simulink model "test_pont_H"  (R2013a)
settings: Solver=ode3  StartTime=0.0  StopTime=1  FixedStep=5e-5  RelTol=1e-3
libraries: powerlib x18, simulink x2, powerlib_meascontrol x2
settings Model: Creator=Daniel  LastModifiedBy=Daniel
settings SolverCC: AlgebraicLoopSolver=LineSearch

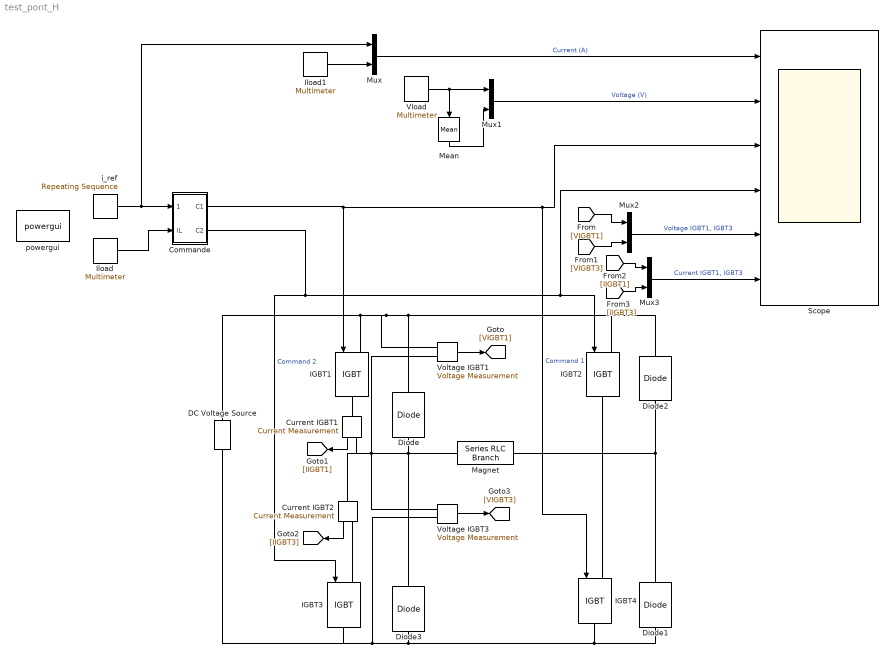
== system test_pont_H ==
  Commande : Subsystem  TreatAsAtomicUnit=on
      settings: MinAlgLoopOccurrences=on
  Current IGBT1 : powerlib/Measurements/Current Measurement  PhasorSimulation=off  OutputType=Complex  PSBequivalent=0
  Current IGBT2 : powerlib/Measurements/Current Measurement  PhasorSimulation=off  OutputType=Complex  PSBequivalent=0
  DC Voltage Source : powerlib/Electrical Sources/DC Voltage Source  Amplitude=5000  Measurements=None
  Diode{,1..3} (4 alike) : powerlib/Power Electronics/Diode  Ron=0.001  Lon=0  Vf=0.8  IC=0  UseSnubber=off  Rs=1  Cs=inf  Measurements=off
  IGBT{1..4} (4 alike) : powerlib/Power Electronics/IGBT  Ron=0.001  Lon=0  Vf=1  Tf=1e-6  Tt=2e-6  IC=0  Rs=0  Cs=0  Measurements=off
  Iload : powerlib/Measurements/Multimeter  PhasorSimulation=off  OutputType=Complex  sel=2  L=2  Gain=1  yselected={'Ib: Magnet '};  PSBOutputType=1  PSBequivalent=0  AxesSetting=[0,0.1,-100,100]  Display=0  SavedBlockNames=-11
  Iload1 : powerlib/Measurements/Multimeter  PhasorSimulation=off  OutputType=Complex  sel=2  L=2  Gain=1  yselected={'Ib: Magnet '};  PSBOutputType=1  PSBequivalent=0  AxesSetting=[0,0.1,-100,100]  Display=0  SavedBlockNames=-11
  "Magnet " : powerlib/Elements/Series RLC Branch  LConnTagsString=__new0  RConnTagsString=__new0  BranchType=RL  Resistance=0.28  Inductance=0.1  SetiL0=off  InitialCurrent=0  Capacitance=1e-6  Setx0=off  InitialVoltage=0  Measurements=Branch voltage and current
  Mean : powerlib_meascontrol/Measurements/Mean  Freq=1e3  Vinit=0  Ts=0
  Mux{,1..3} (4 alike) : Mux  Inputs=2
  Scope : Scope  NumInputPorts=6
      settings: YMin=0~-12500~0~0~-5~-5  YMax=2500~7500~1~1~5~5
  Vload : powerlib/Measurements/Multimeter  PhasorSimulation=off  OutputType=Complex  sel=1  L=2  Gain=1  yselected={'Ub: Magnet '};  PSBOutputType=1  PSBequivalent=0  AxesSetting=[0,0.1,-100,100]  Display=0  SavedBlockNames=-11
  Voltage IGBT1 : powerlib/Measurements/Voltage Measurement  PhasorSimulation=off  OutputType=Complex  PSBequivalent=0
  Voltage IGBT3 : powerlib/Measurements/Voltage Measurement  PhasorSimulation=off  OutputType=Complex  PSBequivalent=0
  "i_ref " : simulink/Sources/Repeating Sequence  rep_seq_t=[0 100e-3 100.1e-3 475e-3 550e-3 708.4e-3 900e-3]  rep_seq_y=[0 0 250 6000 6000 250 250]
  powergui : powerlib/powergui  Priority=1  SimulationMode=Discrete  SolverType=Tustin  SampleTime=50e-6  frequency=60  SPID=off  DisableSnubberDevices=off  DisableRonSwitches=off  DisableVfSwitches=off  SwTol=0  Interpol=off  DisplayEquations=off  frequencyindice=0  Pbase=100e6  ErrMax=1e-4  Iterations=50  UnitsV=kV  UnitsW=MW  FunctionMessages=off  echomessages=off  HookPort=off  EnableUseOfTLC=off  x0status=blocks  RestoreLinks=warning  ResistiveCurrentMeasurement=off  Frange=[0:2:500]  Ylog=off  Xlog=on  ShowGrid=off  save=off  variable=ZData  ZoomFFT=off  StartTime=0.0  cycles=1  DisplayStyle=1  fundamental=60  FreqAxis=off  MaxFrequency=1000  frequencyindicesteady=1  RmsSteady=1  display=off  Ts=0  methode=off
  wires:
  Iload/1 -> Commande/2(IL)
  Commande/1(C1) -> IGBT1/1, IGBT4/1, Scope/3  "Command 1"
  Commande/2(C2) -> IGBT3/1, IGBT2/1, Scope/4  "Command 2"
  Iload1/1 -> Mux/2
  Mux/1 -> Scope/1  "Current (A)"
  Mux1/1 -> Scope/2  "Voltage (V)"
  Vload/1 -> Mean/1, Mux1/1
  Mean/1 -> Mux1/2
  "i_ref "/1 -> Mux/1, Commande/1(Iref)
  Voltage IGBT1/1 -> [VIGBT1]
  Voltage IGBT3/1 -> [VIGBT3]
  [VIGBT1] -> Mux2/1
  [IIGBT1] -> Mux3/1
  [IIGBT3] -> Mux3/2
  Mux2/1 -> Scope/5  "Voltage IGBT1, IGBT3"
  Mux3/1 -> Scope/6  "Current IGBT1, IGBT3"
  Current IGBT1/1 -> [IIGBT1]
  Current IGBT2/1 -> [IIGBT3]
  [VIGBT3] -> Mux2/2
  connections:
  Diode/LConn1 -- Voltage IGBT1/LConn2 -- Current IGBT2/LConn1 -- Current IGBT1/RConn1 -- Voltage IGBT3/LConn1 -- "Magnet "/LConn1 -- Diode3/RConn1
  DC Voltage Source/RConn1 -- IGBT1/LConn1 -- IGBT2/LConn1 -- Diode2/RConn1 -- Diode/RConn1 -- Voltage IGBT1/LConn1
  Diode1/LConn1 -- IGBT4/RConn1 -- Voltage IGBT3/LConn2 -- IGBT3/RConn1 -- DC Voltage Source/LConn1 -- Diode3/LConn1
  Diode1/RConn1 -- Diode2/LConn1 -- IGBT4/LConn1 -- IGBT2/RConn1 -- "Magnet "/RConn1
  IGBT1/RConn1 -- Current IGBT1/LConn1
  IGBT3/LConn1 -- Current IGBT2/RConn1

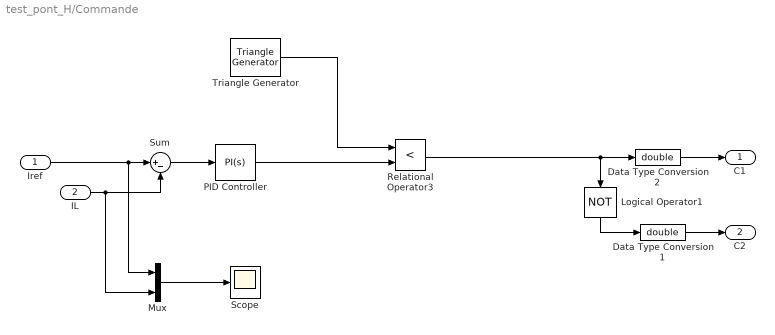
== system test_pont_H/Commande ==
  Iref : Inport
  IL : Inport  Port=2
  Data Type Conversion1 : DataTypeConversion  OutDataTypeStr=double
  Data Type Conversion2 : DataTypeConversion  OutDataTypeStr=double
  Logical Operator1 : Logic  Operator=NOT  AllPortsSameDT=off  OutDataTypeStr=boolean
  Mux : Mux  Inputs=2
  PID Controller : simulink/Continuous/PID Controller  Controller=PI  TimeDomain=Continuous-time  SampleTime=1  IntegratorMethod=Forward Euler  FilterMethod=Forward Euler  Form=Parallel  P=1.12  I=2.8  D=0  N=100  InitialConditionSource=internal  InitialConditionForIntegrator=0  InitialConditionForFilter=0  ExternalReset=none  LimitOutput=on  UpperSaturationLimit=0.95  LowerSaturationLimit=-0.95  LinearizeAsGain=on  AntiWindupMode=clamping  Kb=1  TrackingMode=off  Kt=1  PParamMin=[]  PParamMax=[]  IParamMin=[]  IParamMax=[]  DParamMin=[]  DParamMax=[]  NParamMin=[]  NParamMax=[]  KbParamMin=[]  KbParamMax=[]  KtParamMin=[]  KtParamMax=[]  POutMin=[]  POutMax=[]  IOutMin=[]  IOutMax=[]  DOutMin=[]  DOutMax=[]  NOutMin=[]  NOutMax=[]  KbOutMin=[]  KbOutMax=[]  KtOutMin=[]  KtOutMax=[]  IntegratorOutMin=[]  IntegratorOutMax=[]  FilterOutMin=[]  FilterOutMax=[]  SumOutMin=[]  SumOutMax=[]  SumI1OutMin=[]  SumI1OutMax=[]  SumI2OutMin=[]  SumI2OutMax=[]  SumI3OutMin=[]  SumI3OutMax=[]  SumDOutMin=[]  SumDOutMax=[]  SaturationOutMin=[]  SaturationOutMax=[]  IntegratorContinuousStateAttributes=''  IntegratorStateMustResolveToSignalObject=off  IntegratorRTWStateStorageClass=Auto  FilterContinuousStateAttributes=''  FilterStateMustResolveToSignalObject=off  FilterRTWStateStorageClass=Auto
  Relational Operator3 : RelationalOperator  Operator=<  OutDataTypeStr=boolean
  Scope : Scope
  Sum : Sum  Inputs=|+-
  Triangle Generator : powerlib_meascontrol/Pulse & Signal Generators/Triangle Generator  Freq=1e3  Phase=180  Ts=5e-5
  C1 : Outport
  C2 : Outport  Port=2
  wires:
  IL/1 -> Mux/2, Sum/2
  Triangle Generator/1 -> Relational Operator3/1
  Sum/1 -> PID Controller/1
  Relational Operator3/1 -> Data Type Conversion2/1, Logical Operator1/1
  Data Type Conversion2/1 -> C1/1
  Logical Operator1/1 -> Data Type Conversion1/1
  Data Type Conversion1/1 -> C2/1
  Mux/1 -> Scope/1
  PID Controller/1 -> Relational Operator3/2
  Iref/1 -> Mux/1, Sum/1
